simulink model "mvdc_trajectory_driver"  (R2018b)
settings: configuration reference "Active" (kept outside this file)
undefined symbols (not defined in the file): P_MVDC_ControllerMode, TUMPathMatchingState
libraries: simulink x1
settings Model: DataDictionary=mvdc_trajectory_driver.sldd  Creator=wischnewski  LastModifiedBy=ge34qer

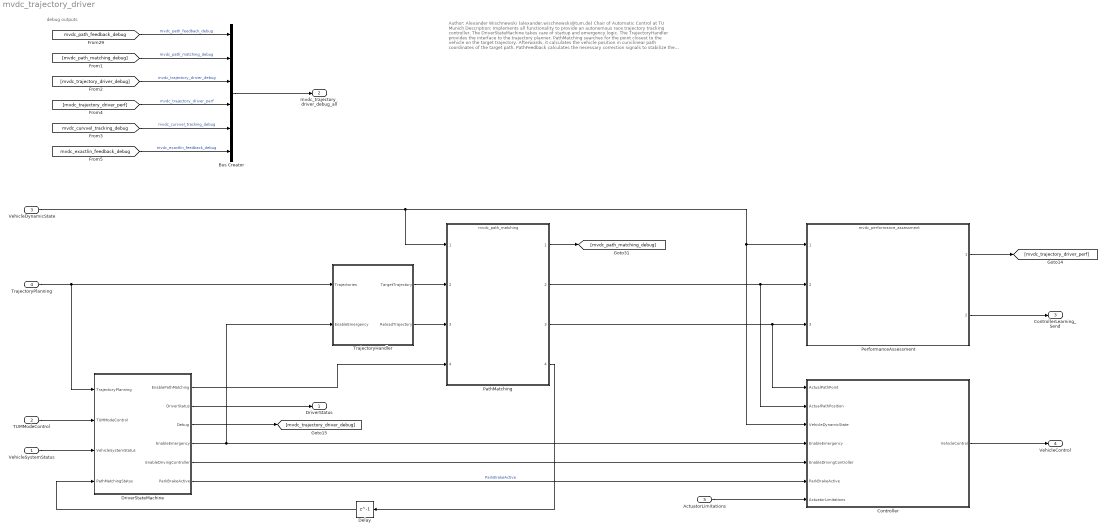
== system mvdc_trajectory_driver ==
  note: debug outputs
  note: Author: Alexander Wischnewski (alexander.wischnewski@tum.de)
      | Chair of Automatic Control at TU Munich
      |
      | Description: Implements all functionality to provide an autonomous race trajectory tracking controller.
      |
      | The DriverStateMachine takes care of startup and emergency logic.
      |
      | The TrajectoryHandler provides the interface to the trajectory planner.
      |
      | PathMatching searches for the point closest to the vehicle on the target trajectory. Afterwards, it calculates
      | the vehicle position in curvilinear path coordinates of the target path.
      |
      | PathFeedback calculates the necessary correction signals to stabilize the vehicle on the target path.
      |
      | PerformanceAssessment evaluates several performance measures and calculates the current lap time.
      |
      | CurvatureVelocityTracking provides a feedback loop for curvature tracking and velocity tracking. Each utilizes
      | a combination of a P-controller with disturbance observer based techniques.
      |
      | Inputs:
      | TUMModeControl Control bits of the vehicle state machine
      | VehicleDynamicState Fused vehicle state vector ( position, velocities, accelerations, etc.)
      | TrajectoryPlanning Inputs from the trajectory planner
      | VehicleSensorData Raw sensor data for all vehicle sesnsors
      |
      | Outputs:
      | DriverStatus Status information about the trajectory tracking controller
      | VehicleControl Low level controller interface of the vehicle
      | ControllerLearning_Send Interface to the controller learning algorithms
  VehicleSystemStatus : Inport  OutDataTypeStr=Bus: VehicleSystemStatus  BusOutputAsStruct=on
  TUMModeControl : Inport  Port=2  OutDataTypeStr=Bus: TUMModeControl  PortDimensions=1  BusOutputAsStruct=on
  VehicleDynamicState : Inport  Port=3  OutDataTypeStr=Bus: VehicleDynamicState
  TrajectoryPlanning : Inport  Port=4  OutDataTypeStr=Bus: TrajectoryPlanning
  ActuatorLimitations : Inport  Port=5  OutDataTypeStr=Bus: ActuatorLimitations  BusOutputAsStruct=on
  Bus Creator : BusCreator  Inputs=6
  Controller : Subsystem
  Delay : Delay  DelayLength=1  InitialCondition=TUMPathMatchingState.PM_OFF
  DriverStateMachine : Subsystem
  PathMatching : ModelReference  ModelNameDialog=mvdc_path_matching  SimulationMode=Normal  ModelReferenceVersion=1.469
  PerformanceAssessment : ModelReference  ModelNameDialog=mvdc_performance_assessment  SimulationMode=Normal  ModelReferenceVersion=1.341
  TrajectoryHandler : Subsystem
  DriverStatus : Outport  OutDataTypeStr=Enum: TUMHealthStatus  PortDimensions=1
  mvdc_trajectory_driver_debug_all : Outport  Port=2  OutDataTypeStr=Bus: mvdc_trajectory_driver_debug_all  PortDimensions=1  BusOutputAsStruct=on
  ControllerLearning_Send : Outport  Port=3  OutDataTypeStr=Bus: ControllerLearning_Send  PortDimensions=1  BusOutputAsStruct=on
  VehicleControl : Outport  Port=4  OutDataTypeStr=Bus: VehicleControl  BusOutputAsStruct=on
  wires:
  PathMatching/2 -> PerformanceAssessment/2, Controller/2(ActualPathPosition)
  PathMatching/3 -> Controller/1(ActualPathPoint), PerformanceAssessment/3
  TUMModeControl/1 -> DriverStateMachine/2(TUMModeControl)
  TrajectoryPlanning/1 -> TrajectoryHandler/1(Trajectories), DriverStateMachine/1(TrajectoryPlanning)
  DriverStateMachine/2(DriverStatus) -> DriverStatus/1
  PathMatching/4 -> Delay/1
  DriverStateMachine/1(EnablePathMatching) -> PathMatching/4
  DriverStateMachine/4(EnableEmergency) -> TrajectoryHandler/2(EnableEmergency), Controller/4(EnableEmergency)
  PathMatching/1 -> [mvdc_path_matching_debug]
  Bus Creator/1 -> mvdc_trajectory_driver_debug_all/1
  DriverStateMachine/3(Debug) -> [mvdc_trajectory_driver_debug]
  PerformanceAssessment/1 -> [mvdc_trajectory_driver_perf]
  [mvdc_path_feedback_debug] -> Bus Creator/1  "mvdc_path_feedback_debug"
  [mvdc_path_matching_debug] -> Bus Creator/2  "mvdc_path_matching_debug"
  [mvdc_trajectory_driver_debug] -> Bus Creator/3  "mvdc_trajectory_driver_debug"
  [mvdc_trajectory_driver_perf] -> Bus Creator/4  "mvdc_trajectory_driver_perf"
  VehicleDynamicState/1 -> PathMatching/1, Controller/3(VehicleDynamicState), PerformanceAssessment/1
  Delay/1 -> DriverStateMachine/4(PathMatchingStatus)
  PerformanceAssessment/2 -> ControllerLearning_Send/1
  [mvdc_curvvel_tracking_debug] -> Bus Creator/5  "mvdc_curvvel_tracking_debug"
  VehicleSystemStatus/1 -> DriverStateMachine/3(VehicleSystemStatus)
  [mvdc_exactlin_feedback_debug] -> Bus Creator/6  "mvdc_exactlin_feedback_debug"
  TrajectoryHandler/1(TargetTrajectory) -> PathMatching/2
  TrajectoryHandler/2(ReloadTrajectory) -> PathMatching/3
  DriverStateMachine/5(EnableDrivingController) -> Controller/5(EnableDrivingController)
  DriverStateMachine/6(ParkBrakeActive) -> Controller/6(ParkBrakeActive)  "ParkBrakeActive"
  ActuatorLimitations/1 -> Controller/7(ActuatorLimitations)
  Controller/1(VehicleControl) -> VehicleControl/1

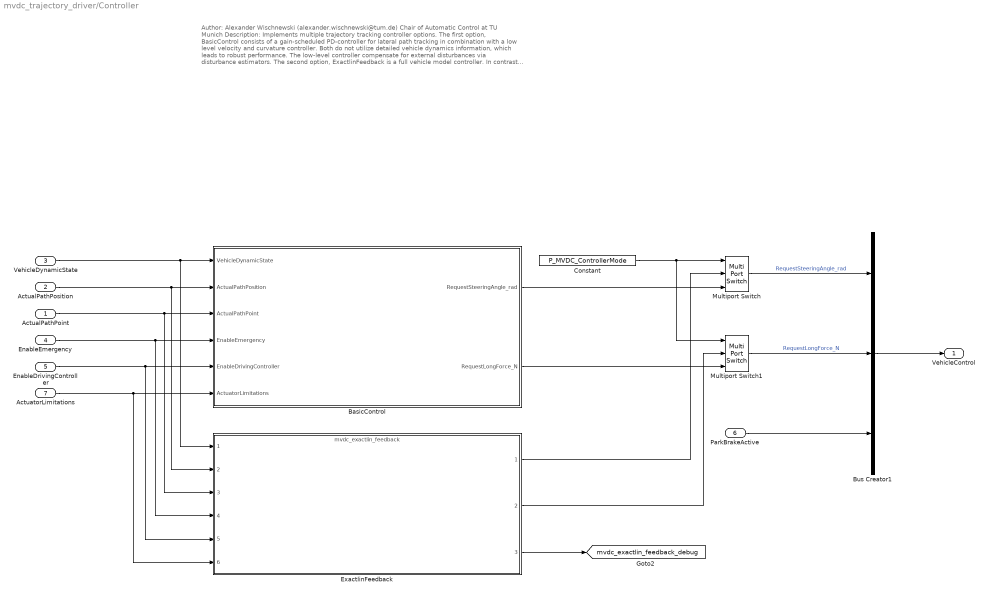
== system mvdc_trajectory_driver/Controller ==
  note: Author: Alexander Wischnewski (alexander.wischnewski@tum.de)
      | Chair of Automatic Control at TU Munich
      |
      | Description: Implements multiple trajectory tracking controller options.
      |
      | The first option, BasicControl consists of a gain-scheduled PD-controller for lateral path tracking in
      | combination with a low level velocity and curvature controller. Both do not utilize detailed vehicle
      | dynamics information, which leads to robust performance. The low-level controller compensate
      | for external disturbances via disturbance estimators.
      |
      | The second option, ExactlinFeedback is a full vehicle model controller. In contrast to classic exact
      | linearization based controllers, it utilizes a steady-state vehicle model. This increases the robustness
      | as it favors steady-state operation in contrast to very agressive feedback control.
      |
      | Inputs:
      | VehicleDynamicState Fused vehicle state vector ( position, velocities, accelerations, etc.)
      | ActualPathPosition Current position in path coordinates
      | ActualPathPoint Current point matched on the target trajectory
      | EnableEmergency Signalize controller that an emergency has been triggered
      | EnableDrivingController Signalize controller that it is allowed to drive now
      | ActuatorLimitations Hardware limitations of the actuators
      |
      | Outputs:
      | VehicleControl Target values for actuators
  ActualPathPoint : Inport
  ActualPathPosition : Inport  Port=2
  VehicleDynamicState : Inport  Port=3
  EnableEmergency : Inport  Port=4  OutDataTypeStr=boolean
  EnableDrivingController : Inport  Port=5
  ParkBrakeActive : Inport  Port=6
  ActuatorLimitations : Inport  Port=7  OutDataTypeStr=Bus: ActuatorLimitations  BusOutputAsStruct=on
  BasicControl : Subsystem
  Bus Creator1 : BusCreator  Inputs=3  OutDataTypeStr=Bus: VehicleControl
      settings: InheritFromInputs=off
  Constant : Constant  Value=P_MVDC_ControllerMode
  ExactlinFeedback : ModelReference  ModelNameDialog=mvdc_exactlin_feedback  SimulationMode=Normal  ModelReferenceVersion=1.1349
  Multiport Switch : MultiPortSwitch  Inputs=2  DiagnosticForDefault=None
  Multiport Switch1 : MultiPortSwitch  Inputs=2  DiagnosticForDefault=None
  VehicleControl : Outport  OutDataTypeStr=Bus: VehicleControl  BusOutputAsStruct=on
  tag scope: mvdc_exactlin_feedback_debug=global
  wires:
  Multiport Switch/1 -> Bus Creator1/1  "RequestSteeringAngle_rad"
  ExactlinFeedback/1 -> Multiport Switch/2
  ParkBrakeActive/1 -> Bus Creator1/3
  Bus Creator1/1 -> VehicleControl/1
  ExactlinFeedback/2 -> Multiport Switch1/2
  ExactlinFeedback/3 -> [mvdc_exactlin_feedback_debug]
  Constant/1 -> Multiport Switch1/1, Multiport Switch/1
  Multiport Switch1/1 -> Bus Creator1/2  "RequestLongForce_N"
  VehicleDynamicState/1 -> ExactlinFeedback/1, BasicControl/1(VehicleDynamicState)
  ActualPathPoint/1 -> ExactlinFeedback/3, BasicControl/3(ActualPathPoint)
  EnableEmergency/1 -> ExactlinFeedback/4, BasicControl/4(EnableEmergency)
  EnableDrivingController/1 -> ExactlinFeedback/5, BasicControl/5(EnableDrivingController)
  ActuatorLimitations/1 -> BasicControl/6(ActuatorLimitations), ExactlinFeedback/6
  BasicControl/1(RequestSteeringAngle_rad) -> Multiport Switch/3
  BasicControl/2(RequestLongForce_N) -> Multiport Switch1/3
  ActualPathPosition/1 -> ExactlinFeedback/2, BasicControl/2(ActualPathPosition)

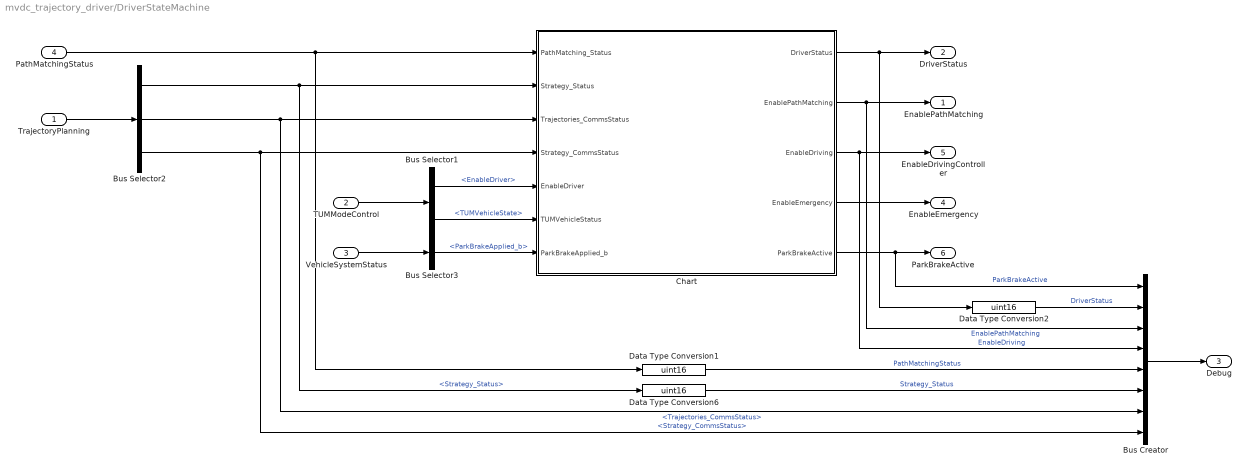
== system mvdc_trajectory_driver/DriverStateMachine ==
  TrajectoryPlanning : Inport  OutDataTypeStr=Bus: TrajectoryPlanning
  TUMModeControl : Inport  Port=2  OutDataTypeStr=Bus: TUMModeControl  PortDimensions=1  BusOutputAsStruct=on
  VehicleSystemStatus : Inport  Port=3  OutDataTypeStr=Bus: VehicleSystemStatus  BusOutputAsStruct=on
  PathMatchingStatus : Inport  Port=4  PortDimensions=1  BusOutputAsStruct=on
  Bus Creator : BusCreator  Inputs=8
  Bus Selector1 : BusSelector  OutputSignals=EnableDriver,TUMVehicleState
  Bus Selector2 : BusSelector  OutputSignals=Strategy_Status,Trajectories_CommsStatus,Strategy_CommsStatus
  Bus Selector3 : BusSelector  OutputSignals=ParkBrakeApplied_b
  Chart : Stateflow chart  TreatAsAtomicUnit=on
  Data Type Conversion1 : DataTypeConversion  OutDataTypeStr=uint16
  Data Type Conversion2 : DataTypeConversion  OutDataTypeStr=uint16
  Data Type Conversion6 : DataTypeConversion  OutDataTypeStr=uint16
  EnablePathMatching : Outport
  DriverStatus : Outport  Port=2  OutDataTypeStr=Enum: TUMHealthStatus  PortDimensions=1
  Debug : Outport  Port=3  OutDataTypeStr=Bus: mvdc_trajectory_driver_debug  PortDimensions=1
  EnableEmergency : Outport  Port=4
  EnableDrivingController : Outport  Port=5
  ParkBrakeActive : Outport  Port=6
  wires:
  Chart/2(EnablePathMatching) -> Bus Creator/3, EnablePathMatching/1  "EnablePathMatching"
  TUMModeControl/1 -> Bus Selector1/1
  Bus Selector1/2 -> Chart/6(TUMVehicleStatus)  "<TUMVehicleState>"
  Bus Selector1/1 -> Chart/5(EnableDriver)  "<EnableDriver>"
  Chart/1(DriverStatus) -> Data Type Conversion2/1, DriverStatus/1
  PathMatchingStatus/1 -> Data Type Conversion1/1, Chart/1(PathMatching_Status)
  TrajectoryPlanning/1 -> Bus Selector2/1
  Bus Selector2/1 -> Data Type Conversion6/1, Chart/2(Strategy_Status)  "<Strategy_Status>"
  Bus Selector2/3 -> Chart/4(Strategy_CommsStatus), Bus Creator/8  "<Strategy_CommsStatus>"
  Bus Selector2/2 -> Bus Creator/7, Chart/3(Trajectories_CommsStatus)  "<Trajectories_CommsStatus>"
  Bus Creator/1 -> Debug/1
  Data Type Conversion6/1 -> Bus Creator/6  "Strategy_Status"
  Data Type Conversion1/1 -> Bus Creator/5  "PathMatchingStatus"
  Data Type Conversion2/1 -> Bus Creator/2  "DriverStatus"
  Chart/3(EnableDriving) -> Bus Creator/4, EnableDrivingController/1  "EnableDriving"
  Chart/4(EnableEmergency) -> EnableEmergency/1
  VehicleSystemStatus/1 -> Bus Selector3/1
  Bus Selector3/1 -> Chart/7(ParkBrakeApplied_b)  "<ParkBrakeApplied_b>"
  Chart/5(ParkBrakeActive) -> Bus Creator/1, ParkBrakeActive/1  "ParkBrakeActive"

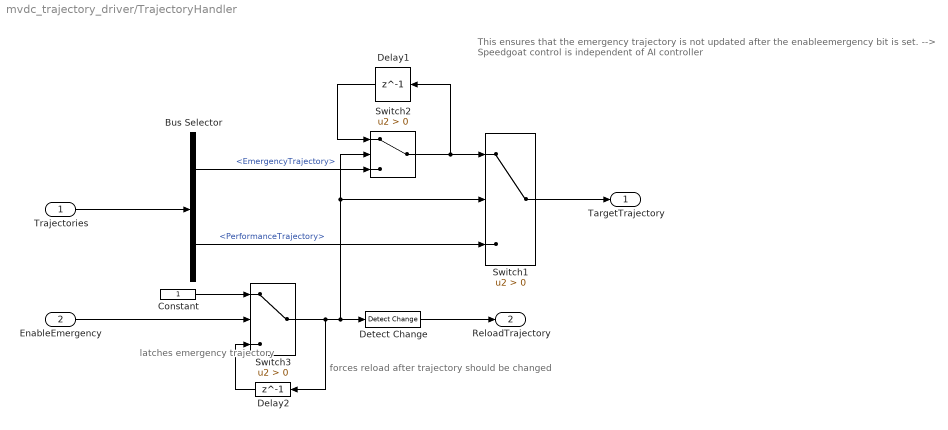
== system mvdc_trajectory_driver/TrajectoryHandler ==
  note: latches emergency
      | trajectory
  note: forces reload after trajectory should be changed
  note: This ensures that the emergency trajectory is not updated after the enableemergency bit is set.
      | --> Speedgoat control is independent of AI controller
  Trajectories : Inport
  EnableEmergency : Inport  Port=2
  Bus Selector : BusSelector  OutputSignals=EmergencyTrajectory,PerformanceTrajectory
  Constant : Constant
  Delay1 : Delay  DelayLength=1
  Delay2 : Delay  DelayLength=1
  Detect Change : simulink/Logic and Bit Operations/Detect Change  vinit=0  OutDataTypeStr=boolean
  Switch1 : Switch  Criteria=u2 > Threshold
  Switch2 : Switch  Criteria=u2 > Threshold
  Switch3 : Switch  Criteria=u2 > Threshold
  TargetTrajectory : Outport
  ReloadTrajectory : Outport  Port=2
  wires:
  Switch2/1 -> Delay1/1, Switch1/1
  Delay1/1 -> Switch2/1
  Trajectories/1 -> Bus Selector/1
  Bus Selector/2 -> Switch1/3  "<PerformanceTrajectory>"
  Switch3/1 -> Delay2/1, Detect Change/1, Switch1/2, Switch2/2
  Bus Selector/1 -> Switch2/3  "<EmergencyTrajectory>"
  Switch1/1 -> TargetTrajectory/1
  Detect Change/1 -> ReloadTrajectory/1
  Delay2/1 -> Switch3/3
  Constant/1 -> Switch3/1
  EnableEmergency/1 -> Switch3/2

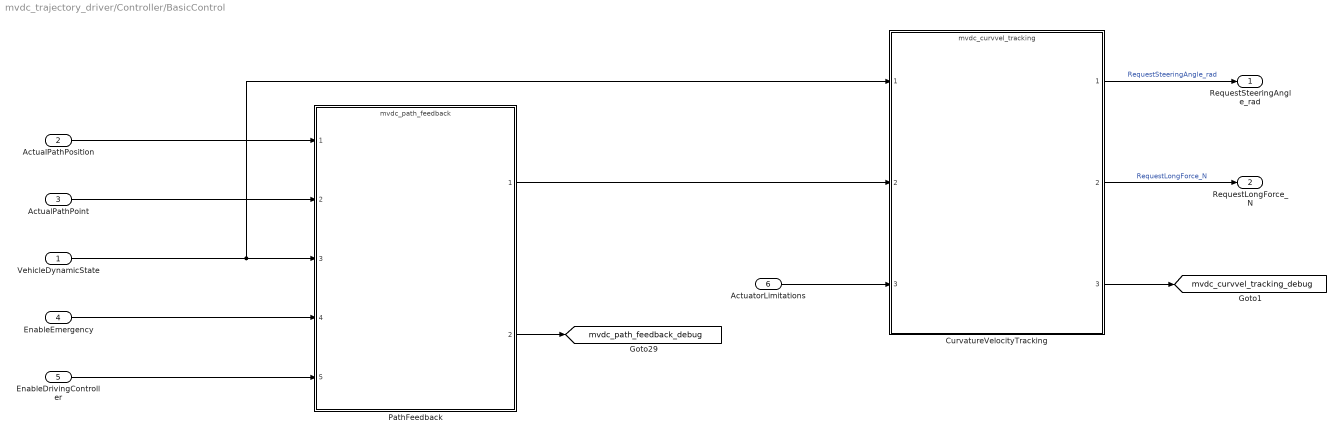
== system mvdc_trajectory_driver/Controller/BasicControl ==
  VehicleDynamicState : Inport
  ActualPathPosition : Inport  Port=2
  ActualPathPoint : Inport  Port=3
  EnableEmergency : Inport  Port=4
  EnableDrivingController : Inport  Port=5
  ActuatorLimitations : Inport  Port=6  OutDataTypeStr=Bus: ActuatorLimitations  BusOutputAsStruct=on
  CurvatureVelocityTracking : ModelReference  ModelNameDialog=mvdc_curvvel_tracking.slx  SimulationMode=Normal  ModelReferenceVersion=1.1219
  PathFeedback : ModelReference  ModelNameDialog=mvdc_path_feedback  SimulationMode=Normal  ModelReferenceVersion=1.630
  RequestSteeringAngle_rad : Outport
  RequestLongForce_N : Outport  Port=2
  tag scope: mvdc_curvvel_tracking_debug=global, mvdc_path_feedback_debug=global
  wires:
  VehicleDynamicState/1 -> CurvatureVelocityTracking/1, PathFeedback/3
  EnableDrivingController/1 -> PathFeedback/5
  ActualPathPoint/1 -> PathFeedback/2
  ActuatorLimitations/1 -> CurvatureVelocityTracking/3
  EnableEmergency/1 -> PathFeedback/4
  PathFeedback/2 -> [mvdc_path_feedback_debug]
  ActualPathPosition/1 -> PathFeedback/1
  CurvatureVelocityTracking/1 -> RequestSteeringAngle_rad/1  "RequestSteeringAngle_rad"
  CurvatureVelocityTracking/2 -> RequestLongForce_N/1  "RequestLongForce_N"
  CurvatureVelocityTracking/3 -> [mvdc_curvvel_tracking_debug]
  PathFeedback/1 -> CurvatureVelocityTracking/2

== stateflow chart mvdc_trajectory_driver/DriverStateMachine/Chart ==
  note: The main purpose of the driver state machine is to handle all functionality
      | regarding the trajectory planner interface and the internals of the path tracking controller.
      |
      | The main states are:
      | DriverPreparing : Checks if trajectories are received, enables path matching and checks if there is a valid match (close enough to the current position)
      | DriverReady2Go : Signalizes the low level vehicle controller that the trajectory tracking controller is ready to go. If the trajectory planner and the low level
      | vehicle interface go to driving, the controller is activated.
      | DriverActive : The controller is fully active, either in normal mode or in emergency mode (differences in low level controller parametrization)
      |
      | The emergency handling is done via the Warning and the Error state. If there is an failure in the controller or in the trajectory planning algorithm which can
      | still be handled via closed-loop controller operation, this should lead to a warning. The vehicle state machine switches the full system to soft emergency in this
      | case but the controller itself stays active. In Error state the vehicle state machine switches to hard emergency which applies brakes as strong as possible.
  state DriverEnabled
    state DriverActive
      state DisablePark
        entry: ParkBrakeActive = false;
      state Emergency
        entry:
        DriverStatus = TUMHealthStatus.WARNING;
        EnableEmergency = true;
      state NormalDriving
        entry:
        EnableDriving = true;
      state ActivatePark
        entry: EnableDriving = false;
        ParkBrakeActive = true;
      (default) -> (junction 29)
      (junction 29) -> DisablePark [order 2]
      (junction 29) -> Emergency [order 1] : [TUMVehicleStatus == EMERGENCY]
      DisablePark -> NormalDriving : [~ParkBrakeApplied_b]
      NormalDriving -> Emergency [order 2] : [PathMatching_Status ~= ...
          | TUMPathMatchingState.PM_VALID || ...
          | (Trajectories_CommsStatus ~= ...
          | TUMHealthStatus.OK) ||...
          | (uint16(Strategy_Status) <...
          | uint16(TUMStrategyState.S_DRIVING_STARTRACE)) ||...
          | (uint16(Strategy_Status) >...
          | uint16(TUMStrategyState.S_DRIVING_BRAKE2STOP)) ||...
          | (Strategy_CommsStatus ~= ...
          | TUMHealthStatus.OK) || ...
          | TUMVehicleStatus == EMERGENCY]
      NormalDriving -> ActivatePark [order 1] : [Strategy_Status == TUMStrategyState.S_STANDSTILL]
    state DriverPreparing
      state DriverReady2Go
        entry:
        DriverStatus = TUMHealthStatus.OK;
      state WaitForPathMatching
        entry:
        EnablePathMatching = true;
      state Standstill
        entry:
        EnableDriving = false;
      (default) -> Standstill
      Standstill -> WaitForPathMatching : after(0.1, sec)
      WaitForPathMatching -> DriverReady2Go : [(PathMatching_Status ==...
          |  TUMPathMatchingState.PM_VALID)]
    (default) -> DriverPreparing
    DriverReady2Go -> DriverActive : [((Strategy_Status ==...
        |  TUMStrategyState.S_DRIVING_STARTRACE) ||...
        | (Strategy_Status ==...
        |  TUMStrategyState.S_DRIVING_RACE)) &&...
        | (TUMVehicleStatus == DRIVING)]
  state WaitForActivation
    entry: DriverStatus = TUMHealthStatus.ERROR;
    ParkBrakeActive = true;
  state Error
    entry:
    DriverStatus = TUMHealthStatus.ERROR;
    EnableDriving = false;
  (default) -> WaitForActivation
  WaitForActivation -> DriverEnabled : [EnableDriver && ...
      | (Strategy_CommsStatus == ...
      | TUMHealthStatus.OK) && ...
      | (Trajectories_CommsStatus == ...
      | TUMHealthStatus.OK)]
  DriverPreparing -> WaitForActivation : [(Strategy_CommsStatus ~= ...
      | TUMHealthStatus.OK) || ...
      | (Trajectories_CommsStatus ~= ...
      | TUMHealthStatus.OK)]
  DriverEnabled -> Error : [~EnableDriver]
  data: PathMatching_Status input Enum: TUMPathMatchingState; Strategy_Status input Enum: TUMStrategyState; Trajectories_CommsStatus input Enum: TUMHealthStatus; Strategy_CommsStatus input Enum: TUMHealthStatus; EnableDriver input boolean; DriverStatus output Enum: TUMHealthStatus =TUMHealthStatus.ERROR; EnablePathMatching output boolean =false; TUMVehicleStatus input Enum: TUMVehicleState; EnableDriving output boolean; EnableEmergency output boolean; ParkBrakeApplied_b input; ParkBrakeActive output
